simulink model "distr_obs_final"  (R2024b)
settings: Solver=VariableStepAuto  StartTime=0.0  StopTime=10  RelTol=1e-3
values from neighbouring files (symbols this model uses):
  A_sta = A-B*K    [main.m]
  Adj = [0,0,0,0,0,0 ... (first row only)    [chain_net.m]    (also in mesh_net.m = [0     3     1     1     1     1; star_net.m)
  C = [708.27 0]    [main.m]
  F = -F    [main.m]
  G = [1,0,0,0,0,0 ... (first row only)    [chain_net.m]    (also in mesh_net.m = diag([1,3,1,2,2,1]); star_net.m)
  noise_freq = 0.1    [main.m]
  noise_level = 10000    [main.m]
  x0 = [10, 1]    [main.m]
  x0_1 = [12 1]    [main.m]
  x0_2 = [4 1]    [main.m]
  x0_3 = [6 1]    [main.m]
  x0_4 = [6 1]    [main.m]
  x0_5 = [9 1]    [main.m]
  x0_6 = [8 1]    [main.m]
undefined symbols (not defined in the file or in its folder): maglev_dyn, observer
libraries: simulink x6
settings Model: Creator=Francesco  LastModifiedBy=filipnykvist

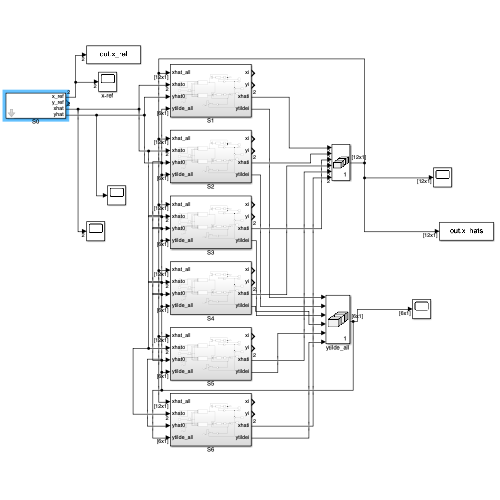
[thumbnail: Simulink's stored preview of the top-level diagram]
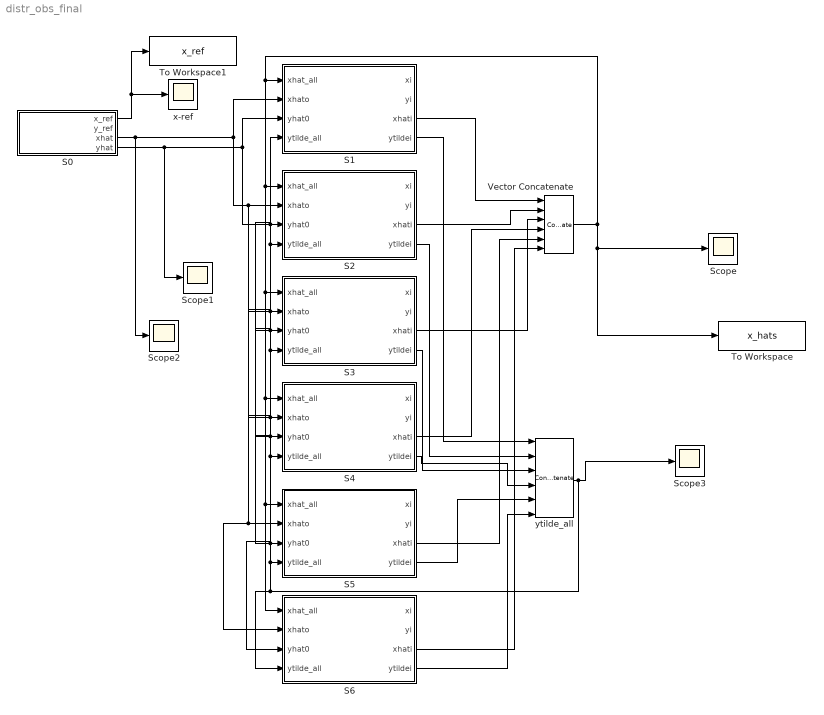
== system distr_obs_final ==
  S0 : Subsystem  mask{node_id=0}
      mask prompts: node_id "Nodo"
  S1 : Subsystem
  S2 : Subsystem
  S3 : Subsystem
  S4 : Subsystem
  S5 : Subsystem
  S6 : Subsystem
  Scope{,1..3} (4 alike) : Scope
  To Workspace : ToWorkspace  VariableName=x_hats  SaveFormat=Timeseries  SampleTime=-1
  To Workspace1 : ToWorkspace  VariableName=x_ref  SaveFormat=Timeseries  SampleTime=-1
  Vector Concatenate : Concatenate  NumInputs=6  Mode=Multidimensional array
  x-ref : Scope
  ytilde_all : Concatenate  NumInputs=6  Mode=Multidimensional array
  wires:
  Vector Concatenate/1 -> To Workspace/1, Scope/1, S6/1(xhat_all), S5/1(xhat_all), S4/1(xhat_all), S3/1(xhat_all), S2/1(xhat_all), S1/1(xhat_all)
  S0/3(xhat) -> Scope2/1, S2/2(xhato), S5/2(xhato), S6/2(xhato), S4/2(xhato), S3/2(xhato), S1/2(xhato)
  ytilde_all/1 -> S1/4(ytilde_all), S2/4(ytilde_all), S3/4(ytilde_all), S4/4(ytilde_all), S5/4(ytilde_all), S6/4(ytilde_all), Scope3/1
  S0/4(yhat) -> Scope1/1, S6/3(yhat0), S5/3(yhat0), S4/3(yhat0), S3/3(yhat0), S2/3(yhat0), S1/3(yhat0)
  S1/3(xhati) -> Vector Concatenate/1
  S2/3(xhati) -> Vector Concatenate/2
  S3/3(xhati) -> Vector Concatenate/3
  S4/3(xhati) -> Vector Concatenate/4
  S5/3(xhati) -> Vector Concatenate/5
  S6/3(xhati) -> Vector Concatenate/6
  S1/4(ytildei) -> ytilde_all/1
  S2/4(ytildei) -> ytilde_all/2
  S3/4(ytildei) -> ytilde_all/3
  S4/4(ytildei) -> ytilde_all/4
  S5/4(ytildei) -> ytilde_all/5
  S6/4(ytildei) -> ytilde_all/6
  S0/1(x_ref) -> x-ref/1, To Workspace1/1

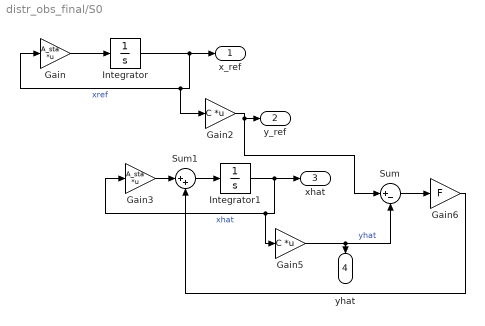
== system distr_obs_final/S0 ==
  Gain : Gain  Gain=A_sta  Multiplication=Matrix(K*u)
  Gain2 : Gain  Gain=C  Multiplication=Matrix(K*u)
  Gain3 : Gain  Gain=A_sta  Multiplication=Matrix(K*u)
  Gain5 : Gain  Gain=C  Multiplication=Matrix(K*u)
  Gain6 : Gain  Gain=F
  Integrator : Integrator  InitialCondition=x0
  Integrator1 : Integrator  InitialCondition=[0,0]'
  Sum : Sum  Inputs=|+-
  Sum1 : Sum  Inputs=|++
  x_ref : Outport
  y_ref : Outport  Port=2
  xhat : Outport  Port=3
  yhat : Outport  Port=4
  wires:
  Gain/1 -> Integrator/1
  Integrator/1 -> Gain/1, Gain2/1, x_ref/1  "xref"
  Gain2/1 -> Sum/1, y_ref/1
  Integrator1/1 -> Gain3/1, Gain5/1, xhat/1  "xhat"
  Gain5/1 -> yhat/1, Sum/2  "yhat"
  Sum/1 -> Gain6/1
  Gain3/1 -> Sum1/1
  Sum1/1 -> Integrator1/1
  Gain6/1 -> Sum1/2

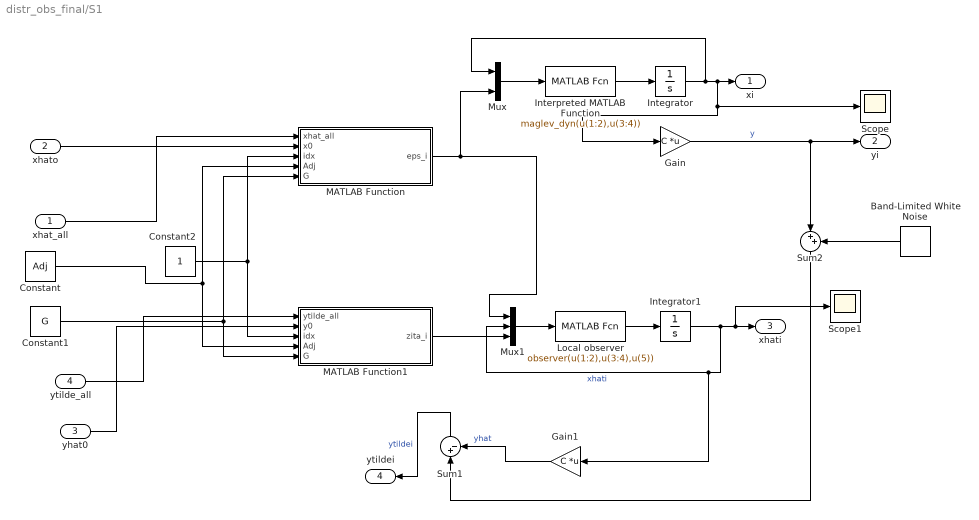
== system distr_obs_final/S1 ==
  xhat_all : Inport
  xhato : Inport  Port=2
  yhat0 : Inport  Port=3
  ytilde_all : Inport  Port=4
  Band-Limited White Noise : simulink/Sources/Band-Limited White Noise  Cov=[noise_level]  Ts=noise_freq  seed=[23341]
  Constant : Constant  Value=Adj
  Constant1 : Constant  Value=G
  Constant2 : Constant
  Gain : Gain  Gain=C  Multiplication=Matrix(K*u)
  Gain1 : Gain  Gain=C  Multiplication=Matrix(K*u)
  Integrator : Integrator  InitialCondition=x0_1
  Integrator1 : Integrator  InitialCondition=[0,0]'
  Interpreted MATLAB Function : MATLABFcn  MATLABFcn=maglev_dyn(u(1:2),u(3:4))
  Local observer : MATLABFcn  MATLABFcn=observer(u(1:2),u(3:4),u(5))  OutputDimensions=2
  MATLAB Function : MATLAB Function  TreatAsAtomicUnit=on
  MATLAB Function1 : MATLAB Function  TreatAsAtomicUnit=on
  Mux : Mux  Inputs=2
  Mux1 : Mux  Inputs=3
  Scope : Scope
  Scope1 : Scope
  Sum1 : Sum  Inputs=|+-
  Sum2 : Sum  Inputs=|++
  xi : Outport
  yi : Outport  Port=2
  xhati : Outport  Port=3
  ytildei : Outport  Port=4
  wires:
  Mux/1 -> Interpreted MATLAB Function/1
  Integrator/1 -> Mux/1, Scope/1, Gain/1, xi/1
  Interpreted MATLAB Function/1 -> Integrator/1
  Gain/1 -> Sum2/1, yi/1  "y"
  Local observer/1 -> Integrator1/1
  Integrator1/1 -> Mux1/2, Gain1/1, Scope1/1, xhati/1  "xhati"
  Gain1/1 -> Sum1/2  "yhat"
  Sum1/1 -> ytildei/1  "ytildei"
  xhat_all/1 -> MATLAB Function/1(xhat_all)
  Constant/1 -> MATLAB Function1/4(Adj), MATLAB Function/4(Adj)
  Constant1/1 -> MATLAB Function1/5(G), MATLAB Function/5(G)
  Constant2/1 -> MATLAB Function1/3(idx), MATLAB Function/3(idx)
  Mux1/1 -> Local observer/1
  MATLAB Function/1(eps_i) -> Mux/2, Mux1/1
  xhato/1 -> MATLAB Function/2(x0)
  Band-Limited White Noise/1 -> Sum2/2
  Sum2/1 -> Sum1/1
  MATLAB Function1/1(zita_i) -> Mux1/3
  ytilde_all/1 -> MATLAB Function1/1(ytilde_all)
  yhat0/1 -> MATLAB Function1/2(y0)

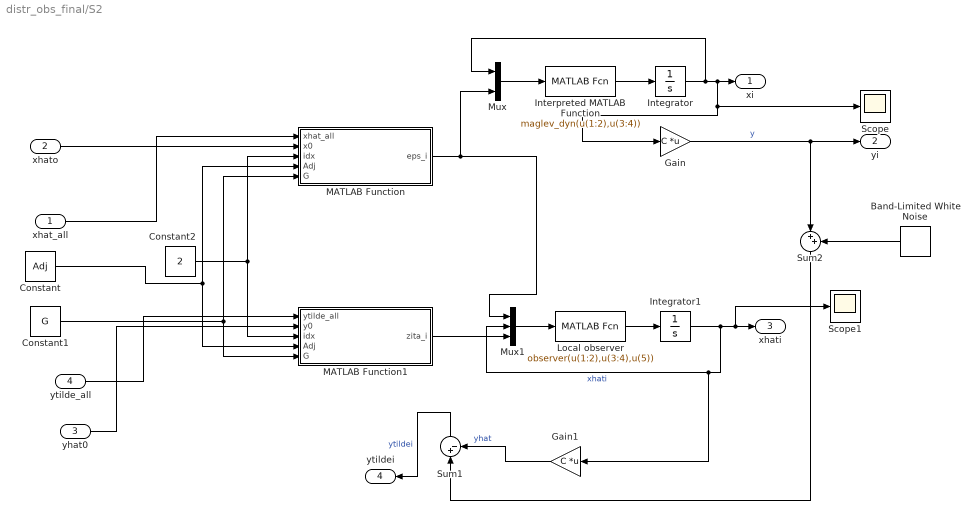
== system distr_obs_final/S2 ==
  xhat_all : Inport
  xhato : Inport  Port=2
  yhat0 : Inport  Port=3
  ytilde_all : Inport  Port=4
  Band-Limited White Noise : simulink/Sources/Band-Limited White Noise  Cov=[noise_level]  Ts=noise_freq  seed=[23341]
  Constant : Constant  Value=Adj
  Constant1 : Constant  Value=G
  Constant2 : Constant  Value=2
  Gain : Gain  Gain=C  Multiplication=Matrix(K*u)
  Gain1 : Gain  Gain=C  Multiplication=Matrix(K*u)
  Integrator : Integrator  InitialCondition=x0_2
  Integrator1 : Integrator  InitialCondition=[0,0]'
  Interpreted MATLAB Function : MATLABFcn  MATLABFcn=maglev_dyn(u(1:2),u(3:4))
  Local observer : MATLABFcn  MATLABFcn=observer(u(1:2),u(3:4),u(5))  OutputDimensions=2
  MATLAB Function : MATLAB Function  TreatAsAtomicUnit=on
  MATLAB Function1 : MATLAB Function  TreatAsAtomicUnit=on
  Mux : Mux  Inputs=2
  Mux1 : Mux  Inputs=3
  Scope : Scope
  Scope1 : Scope
  Sum1 : Sum  Inputs=|+-
  Sum2 : Sum  Inputs=|++
  xi : Outport
  yi : Outport  Port=2
  xhati : Outport  Port=3
  ytildei : Outport  Port=4
  wires:
  Mux/1 -> Interpreted MATLAB Function/1
  Integrator/1 -> Mux/1, Scope/1, Gain/1, xi/1
  Interpreted MATLAB Function/1 -> Integrator/1
  Gain/1 -> Sum2/1, yi/1  "y"
  Local observer/1 -> Integrator1/1
  Integrator1/1 -> Mux1/2, Gain1/1, Scope1/1, xhati/1  "xhati"
  Gain1/1 -> Sum1/2  "yhat"
  Sum1/1 -> ytildei/1  "ytildei"
  xhat_all/1 -> MATLAB Function/1(xhat_all)
  Constant/1 -> MATLAB Function1/4(Adj), MATLAB Function/4(Adj)
  Constant1/1 -> MATLAB Function1/5(G), MATLAB Function/5(G)
  Constant2/1 -> MATLAB Function1/3(idx), MATLAB Function/3(idx)
  Mux1/1 -> Local observer/1
  MATLAB Function/1(eps_i) -> Mux/2, Mux1/1
  xhato/1 -> MATLAB Function/2(x0)
  Band-Limited White Noise/1 -> Sum2/2
  Sum2/1 -> Sum1/1
  MATLAB Function1/1(zita_i) -> Mux1/3
  ytilde_all/1 -> MATLAB Function1/1(ytilde_all)
  yhat0/1 -> MATLAB Function1/2(y0)

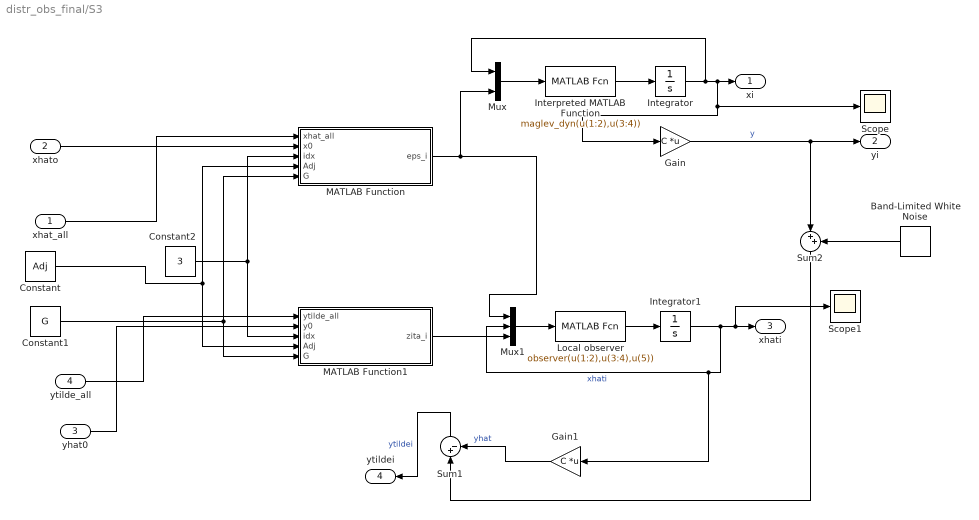
== system distr_obs_final/S3 ==
  xhat_all : Inport
  xhato : Inport  Port=2
  yhat0 : Inport  Port=3
  ytilde_all : Inport  Port=4
  Band-Limited White Noise : simulink/Sources/Band-Limited White Noise  Cov=[noise_level]  Ts=noise_freq  seed=[23341]
  Constant : Constant  Value=Adj
  Constant1 : Constant  Value=G
  Constant2 : Constant  Value=3
  Gain : Gain  Gain=C  Multiplication=Matrix(K*u)
  Gain1 : Gain  Gain=C  Multiplication=Matrix(K*u)
  Integrator : Integrator  InitialCondition=x0_3
  Integrator1 : Integrator  InitialCondition=[0,0]'
  Interpreted MATLAB Function : MATLABFcn  MATLABFcn=maglev_dyn(u(1:2),u(3:4))
  Local observer : MATLABFcn  MATLABFcn=observer(u(1:2),u(3:4),u(5))  OutputDimensions=2
  MATLAB Function : MATLAB Function  TreatAsAtomicUnit=on
  MATLAB Function1 : MATLAB Function  TreatAsAtomicUnit=on
  Mux : Mux  Inputs=2
  Mux1 : Mux  Inputs=3
  Scope : Scope
  Scope1 : Scope
  Sum1 : Sum  Inputs=|+-
  Sum2 : Sum  Inputs=|++
  xi : Outport
  yi : Outport  Port=2
  xhati : Outport  Port=3
  ytildei : Outport  Port=4
  wires:
  Mux/1 -> Interpreted MATLAB Function/1
  Integrator/1 -> Mux/1, Scope/1, Gain/1, xi/1
  Interpreted MATLAB Function/1 -> Integrator/1
  Gain/1 -> Sum2/1, yi/1  "y"
  Local observer/1 -> Integrator1/1
  Integrator1/1 -> Mux1/2, Gain1/1, Scope1/1, xhati/1  "xhati"
  Gain1/1 -> Sum1/2  "yhat"
  Sum1/1 -> ytildei/1  "ytildei"
  xhat_all/1 -> MATLAB Function/1(xhat_all)
  Constant/1 -> MATLAB Function1/4(Adj), MATLAB Function/4(Adj)
  Constant1/1 -> MATLAB Function1/5(G), MATLAB Function/5(G)
  Constant2/1 -> MATLAB Function1/3(idx), MATLAB Function/3(idx)
  Mux1/1 -> Local observer/1
  MATLAB Function/1(eps_i) -> Mux/2, Mux1/1
  xhato/1 -> MATLAB Function/2(x0)
  Band-Limited White Noise/1 -> Sum2/2
  Sum2/1 -> Sum1/1
  MATLAB Function1/1(zita_i) -> Mux1/3
  ytilde_all/1 -> MATLAB Function1/1(ytilde_all)
  yhat0/1 -> MATLAB Function1/2(y0)

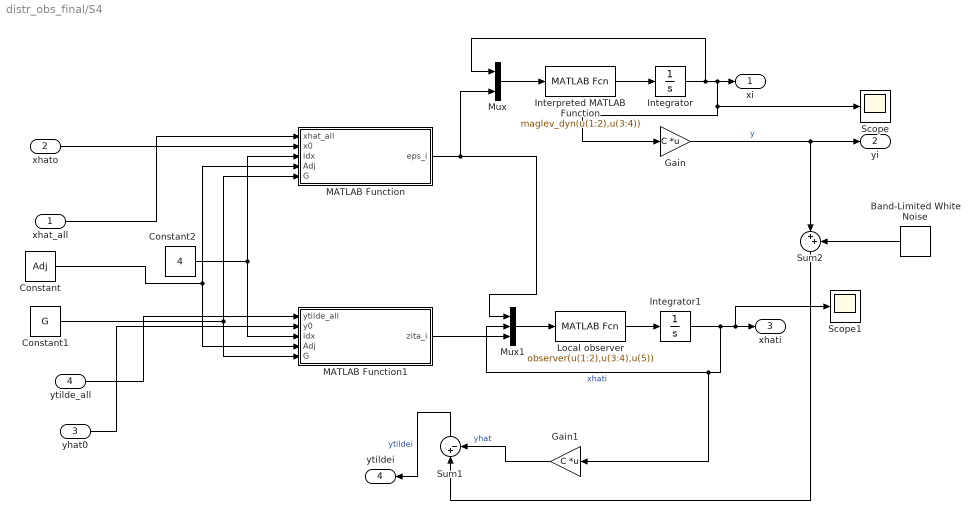
== system distr_obs_final/S4 ==
  xhat_all : Inport
  xhato : Inport  Port=2
  yhat0 : Inport  Port=3
  ytilde_all : Inport  Port=4
  Band-Limited White Noise : simulink/Sources/Band-Limited White Noise  Cov=[noise_level]  Ts=noise_freq  seed=[23341]
  Constant : Constant  Value=Adj
  Constant1 : Constant  Value=G
  Constant2 : Constant  Value=4
  Gain : Gain  Gain=C  Multiplication=Matrix(K*u)
  Gain1 : Gain  Gain=C  Multiplication=Matrix(K*u)
  Integrator : Integrator  InitialCondition=x0_4
  Integrator1 : Integrator  InitialCondition=[0,0]'
  Interpreted MATLAB Function : MATLABFcn  MATLABFcn=maglev_dyn(u(1:2),u(3:4))
  Local observer : MATLABFcn  MATLABFcn=observer(u(1:2),u(3:4),u(5))  OutputDimensions=2
  MATLAB Function : MATLAB Function  TreatAsAtomicUnit=on
  MATLAB Function1 : MATLAB Function  TreatAsAtomicUnit=on
  Mux : Mux  Inputs=2
  Mux1 : Mux  Inputs=3
  Scope : Scope
  Scope1 : Scope
  Sum1 : Sum  Inputs=|+-
  Sum2 : Sum  Inputs=|++
  xi : Outport
  yi : Outport  Port=2
  xhati : Outport  Port=3
  ytildei : Outport  Port=4
  wires:
  Mux/1 -> Interpreted MATLAB Function/1
  Integrator/1 -> Mux/1, Scope/1, Gain/1, xi/1
  Interpreted MATLAB Function/1 -> Integrator/1
  Gain/1 -> Sum2/1, yi/1  "y"
  Local observer/1 -> Integrator1/1
  Integrator1/1 -> Mux1/2, Gain1/1, Scope1/1, xhati/1  "xhati"
  Gain1/1 -> Sum1/2  "yhat"
  Sum1/1 -> ytildei/1  "ytildei"
  xhat_all/1 -> MATLAB Function/1(xhat_all)
  Constant/1 -> MATLAB Function1/4(Adj), MATLAB Function/4(Adj)
  Constant1/1 -> MATLAB Function1/5(G), MATLAB Function/5(G)
  Constant2/1 -> MATLAB Function1/3(idx), MATLAB Function/3(idx)
  Mux1/1 -> Local observer/1
  MATLAB Function/1(eps_i) -> Mux/2, Mux1/1
  xhato/1 -> MATLAB Function/2(x0)
  Band-Limited White Noise/1 -> Sum2/2
  Sum2/1 -> Sum1/1
  MATLAB Function1/1(zita_i) -> Mux1/3
  ytilde_all/1 -> MATLAB Function1/1(ytilde_all)
  yhat0/1 -> MATLAB Function1/2(y0)

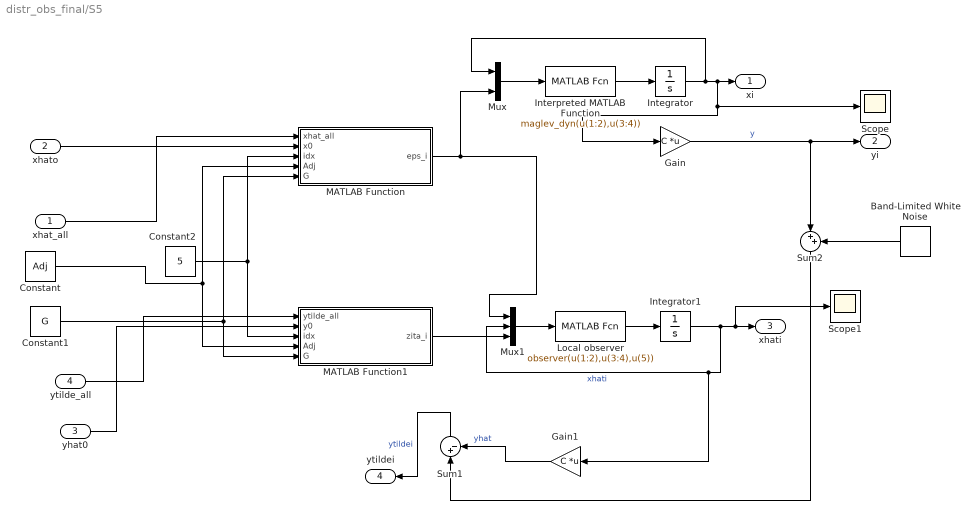
== system distr_obs_final/S5 ==
  xhat_all : Inport
  xhato : Inport  Port=2
  yhat0 : Inport  Port=3
  ytilde_all : Inport  Port=4
  Band-Limited White Noise : simulink/Sources/Band-Limited White Noise  Cov=[noise_level]  Ts=noise_freq  seed=[23341]
  Constant : Constant  Value=Adj
  Constant1 : Constant  Value=G
  Constant2 : Constant  Value=5
  Gain : Gain  Gain=C  Multiplication=Matrix(K*u)
  Gain1 : Gain  Gain=C  Multiplication=Matrix(K*u)
  Integrator : Integrator  InitialCondition=x0_5
  Integrator1 : Integrator  InitialCondition=[0,0]'
  Interpreted MATLAB Function : MATLABFcn  MATLABFcn=maglev_dyn(u(1:2),u(3:4))
  Local observer : MATLABFcn  MATLABFcn=observer(u(1:2),u(3:4),u(5))  OutputDimensions=2
  MATLAB Function : MATLAB Function  TreatAsAtomicUnit=on
  MATLAB Function1 : MATLAB Function  TreatAsAtomicUnit=on
  Mux : Mux  Inputs=2
  Mux1 : Mux  Inputs=3
  Scope : Scope
  Scope1 : Scope
  Sum1 : Sum  Inputs=|+-
  Sum2 : Sum  Inputs=|++
  xi : Outport
  yi : Outport  Port=2
  xhati : Outport  Port=3
  ytildei : Outport  Port=4
  wires:
  Mux/1 -> Interpreted MATLAB Function/1
  Integrator/1 -> Mux/1, Scope/1, Gain/1, xi/1
  Interpreted MATLAB Function/1 -> Integrator/1
  Gain/1 -> Sum2/1, yi/1  "y"
  Local observer/1 -> Integrator1/1
  Integrator1/1 -> Mux1/2, Gain1/1, Scope1/1, xhati/1  "xhati"
  Gain1/1 -> Sum1/2  "yhat"
  Sum1/1 -> ytildei/1  "ytildei"
  xhat_all/1 -> MATLAB Function/1(xhat_all)
  Constant/1 -> MATLAB Function1/4(Adj), MATLAB Function/4(Adj)
  Constant1/1 -> MATLAB Function1/5(G), MATLAB Function/5(G)
  Constant2/1 -> MATLAB Function1/3(idx), MATLAB Function/3(idx)
  Mux1/1 -> Local observer/1
  MATLAB Function/1(eps_i) -> Mux/2, Mux1/1
  xhato/1 -> MATLAB Function/2(x0)
  Band-Limited White Noise/1 -> Sum2/2
  Sum2/1 -> Sum1/1
  MATLAB Function1/1(zita_i) -> Mux1/3
  ytilde_all/1 -> MATLAB Function1/1(ytilde_all)
  yhat0/1 -> MATLAB Function1/2(y0)

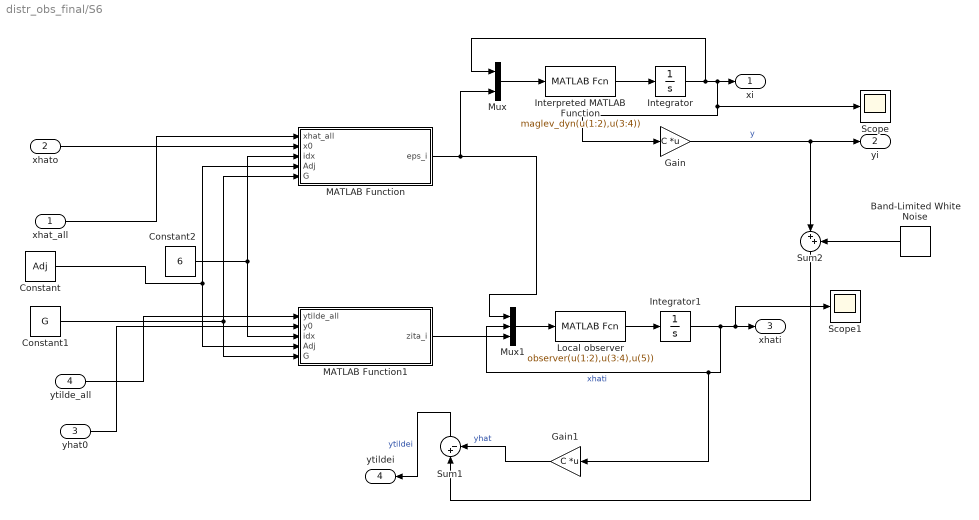
== system distr_obs_final/S6 ==
  xhat_all : Inport
  xhato : Inport  Port=2
  yhat0 : Inport  Port=3
  ytilde_all : Inport  Port=4
  Band-Limited White Noise : simulink/Sources/Band-Limited White Noise  Cov=[noise_level]  Ts=noise_freq  seed=[23341]
  Constant : Constant  Value=Adj
  Constant1 : Constant  Value=G
  Constant2 : Constant  Value=6
  Gain : Gain  Gain=C  Multiplication=Matrix(K*u)
  Gain1 : Gain  Gain=C  Multiplication=Matrix(K*u)
  Integrator : Integrator  InitialCondition=x0_6
  Integrator1 : Integrator  InitialCondition=[0,0]'
  Interpreted MATLAB Function : MATLABFcn  MATLABFcn=maglev_dyn(u(1:2),u(3:4))
  Local observer : MATLABFcn  MATLABFcn=observer(u(1:2),u(3:4),u(5))  OutputDimensions=2
  MATLAB Function : MATLAB Function  TreatAsAtomicUnit=on
  MATLAB Function1 : MATLAB Function  TreatAsAtomicUnit=on
  Mux : Mux  Inputs=2
  Mux1 : Mux  Inputs=3
  Scope : Scope
  Scope1 : Scope
  Sum1 : Sum  Inputs=|+-
  Sum2 : Sum  Inputs=|++
  xi : Outport
  yi : Outport  Port=2
  xhati : Outport  Port=3
  ytildei : Outport  Port=4
  wires:
  Mux/1 -> Interpreted MATLAB Function/1
  Integrator/1 -> Mux/1, Scope/1, Gain/1, xi/1
  Interpreted MATLAB Function/1 -> Integrator/1
  Gain/1 -> Sum2/1, yi/1  "y"
  Local observer/1 -> Integrator1/1
  Integrator1/1 -> Mux1/2, Gain1/1, Scope1/1, xhati/1  "xhati"
  Gain1/1 -> Sum1/2  "yhat"
  Sum1/1 -> ytildei/1  "ytildei"
  xhat_all/1 -> MATLAB Function/1(xhat_all)
  Constant/1 -> MATLAB Function1/4(Adj), MATLAB Function/4(Adj)
  Constant1/1 -> MATLAB Function1/5(G), MATLAB Function/5(G)
  Constant2/1 -> MATLAB Function1/3(idx), MATLAB Function/3(idx)
  Mux1/1 -> Local observer/1
  MATLAB Function/1(eps_i) -> Mux/2, Mux1/1
  xhato/1 -> MATLAB Function/2(x0)
  Band-Limited White Noise/1 -> Sum2/2
  Sum2/1 -> Sum1/1
  MATLAB Function1/1(zita_i) -> Mux1/3
  ytilde_all/1 -> MATLAB Function1/1(ytilde_all)
  yhat0/1 -> MATLAB Function1/2(y0)

== matlab function distr_obs_final/S2/MATLAB Function ==
  data: xhat_all input; eps_i output; x0 input; idx input; Adj input; G input
function eps_i = calcola_epsilon(xhat_all, x0, idx, Adj, G)
    
    a_row = Adj(idx, :);
    g_row = G(idx, :);

    % Assicurazione che i vettori siano nelle giuste forme  
    x0 = x0(:);            
    xhat_all = xhat_all(:); 

    % Selezione del blocco 2x1 corrente
    idx_i = 2 * idx - 1;                      
    xhat_i = xhat_all(idx_i : idx_i + 1);      
                 
    g_i = g_row(idx);                      

    % Dimensioni
    nCols = length(a_row); % nCols = 6
    
    % Inizializzazione matrice estesa a blocchi
    a_row_expand = zeros(2, 2 * nCols); % 2x12

    % Costruzione della matrixe estesa
    for c = 1 : nCols 
        val = a_row(1, c);
        colPos = 2 * c - 1;
        if val ~= 0
            a_row_expand(:, colPos:colPos+1) = val * eye(2);
        end
    end

    % Differenze
    xdiff = xhat_all - repmat(xhat_i, nCols, 1);  
    xdiff = reshape(xdiff, 12, 1);                 
    diff_ref = x0 - xhat_i;                      

    % Calcolo eps_i
    eps_i = a_row_expand * xdiff + g_i * diff_ref;  % 2x1
end

== matlab function distr_obs_final/S5/MATLAB Function1 ==
  data: ytilde_all input; zita_i output; y0 input; idx input; Adj input; G input
function zita_i = calcola_zita(ytilde_all, y0, idx, Adj, G)
    % Get adjacency and pinning row for agent i.
    a_row = Adj(idx, :);
    g_i = G(idx, idx);  

    % Extract ytilde_i.
    ytilde_i = ytilde_all(idx);

    % Compute the difference to each neighbor.
    ydiff = ytilde_all - ytilde_i;  % 6x1 vector of differences

    % Weighted sum of neighbor differences.
    sum_neighbors = a_row * ydiff;  % scalar

    % Leader (reference) difference.
    diff_ref = y0 - ytilde_i;       % scalar

    % Combine to form zita_i.
    zita_i = sum_neighbors + g_i * diff_ref;  % scalar
end

== matlab function distr_obs_final/S6/MATLAB Function ==
  data: xhat_all input; eps_i output; x0 input; idx input; Adj input; G input
function eps_i = calcola_epsilon(xhat_all, x0, idx, Adj, G)
    
    a_row = Adj(idx, :);
    g_row = G(idx, :);

    % Assicurazione che i vettori siano nelle giuste forme  
    x0 = x0(:);            
    xhat_all = xhat_all(:); 

    % Selezione del blocco 2x1 corrente
    idx_i = 2 * idx - 1;                      
    xhat_i = xhat_all(idx_i : idx_i + 1);      
                 
    g_i = g_row(idx);                      

    % Dimensioni
    nCols = length(a_row); % nCols = 6
    
    % Inizializzazione matrice estesa a blocchi
    a_row_expand = zeros(2, 2 * nCols); % 2x12

    % Costruzione della matrixe estesa
    for c = 1 : nCols 
        val = a_row(1, c);
        colPos = 2 * c - 1;
        if val ~= 0
            a_row_expand(:, colPos:colPos+1) = val * eye(2);
        end
    end

    % Differenze
    xdiff = xhat_all - repmat(xhat_i, nCols, 1);  
    xdiff = reshape(xdiff, 12, 1);                 
    diff_ref = x0 - xhat_i;                      

    % Calcolo eps_i
    eps_i = a_row_expand * xdiff + g_i * diff_ref;  % 2x1
end

== matlab function distr_obs_final/S6/MATLAB Function1 ==
  data: ytilde_all input; zita_i output; y0 input; idx input; Adj input; G input
function zita_i = calcola_zita(ytilde_all, y0, idx, Adj, G)
    % Get adjacency and pinning row for agent i.
    a_row = Adj(idx, :);
    g_i = G(idx, idx); 

    % Extract ytilde_i.
    ytilde_i = ytilde_all(idx);

    % Compute the difference to each neighbor.
    ydiff = ytilde_all - ytilde_i;  % 6x1 vector of differences

    % Weighted sum of neighbor differences.
    sum_neighbors = a_row * ydiff;  % scalar

    % Leader (reference) difference.
    diff_ref = y0 - ytilde_i;       % scalar

    % Combine to form zita_i.
    zita_i = sum_neighbors + g_i * diff_ref;  % scalar
end

== matlab function distr_obs_final/S1/MATLAB Function ==
  data: xhat_all input; eps_i output; x0 input; idx input; Adj input; G input
function eps_i = calcola_epsilon(xhat_all, x0, idx, Adj, G)
    
    a_row = Adj(idx, :);
    g_row = G(idx, :);

    % Assicurazione che i vettori siano nelle giuste forme  
    x0 = x0(:);            
    xhat_all = xhat_all(:); 

    % Selezione del blocco 2x1 corrente
    idx_i = 2 * idx - 1;                      
    xhat_i = xhat_all(idx_i : idx_i + 1);      
                 
    g_i = g_row(idx);                      

    % Dimensioni
    nCols = length(a_row); % nCols = 6
    
    % Inizializzazione matrice estesa a blocchi
    a_row_expand = zeros(2, 2 * nCols); % 2x12

    % Costruzione della matrixe estesa
    for c = 1 : nCols 
        val = a_row(1, c);
        colPos = 2 * c - 1;
        if val ~= 0
            a_row_expand(:, colPos:colPos+1) = val * eye(2);
        end
    end

    % Differenze
    xdiff = xhat_all - repmat(xhat_i, nCols, 1);  
    xdiff = reshape(xdiff, 12, 1);                 
    diff_ref = x0 - xhat_i;                      

    % Calcolo eps_i
    eps_i = a_row_expand * xdiff + g_i * diff_ref;  % 2x1
end

== matlab function distr_obs_final/S2/MATLAB Function1 ==
  data: ytilde_all input; zita_i output; y0 input; idx input; Adj input; G input
function zita_i = calcola_zita(ytilde_all, y0, idx, Adj, G)
    % Get adjacency and pinning row for agent i.
    a_row = Adj(idx, :);
    g_i = G(idx, idx);

    % Extract ytilde_i.
    ytilde_i = ytilde_all(idx);

    % Compute the difference to each neighbor.
    ydiff = ytilde_all - ytilde_i;  % 6x1 vector of differences

    % Weighted sum of neighbor differences.
    sum_neighbors = a_row * ydiff;  % scalar

    % Leader (reference) difference.
    diff_ref = y0 - ytilde_i;       % scalar

    % Combine to form zita_i.
    zita_i = sum_neighbors + g_i * diff_ref;  % scalar
end

== matlab function distr_obs_final/S3/MATLAB Function ==
  data: xhat_all input; eps_i output; x0 input; idx input; Adj input; G input
function eps_i = calcola_epsilon(xhat_all, x0, idx, Adj, G)
    
    a_row = Adj(idx, :);
    g_row = G(idx, :);

    % Assicurazione che i vettori siano nelle giuste forme  
    x0 = x0(:);            
    xhat_all = xhat_all(:); 

    % Selezione del blocco 2x1 corrente
    idx_i = 2 * idx - 1;                      
    xhat_i = xhat_all(idx_i : idx_i + 1);      
                 
    g_i = g_row(idx);                      

    % Dimensioni
    nCols = length(a_row); % nCols = 6
    
    % Inizializzazione matrice estesa a blocchi
    a_row_expand = zeros(2, 2 * nCols); % 2x12

    % Costruzione della matrixe estesa
    for c = 1 : nCols 
        val = a_row(1, c);
        colPos = 2 * c - 1;
        if val ~= 0
            a_row_expand(:, colPos:colPos+1) = val * eye(2);
        end
    end

    % Differenze
    xdiff = xhat_all - repmat(xhat_i, nCols, 1);  
    xdiff = reshape(xdiff, 12, 1);                 
    diff_ref = x0 - xhat_i;                      

    % Calcolo eps_i
    eps_i = a_row_expand * xdiff + g_i * diff_ref;  % 2x1
end

== matlab function distr_obs_final/S3/MATLAB Function1 ==
  data: ytilde_all input; zita_i output; y0 input; idx input; Adj input; G input
function zita_i = calcola_zita(ytilde_all, y0, idx, Adj, G)
    % Get adjacency and pinning row for agent i.
    a_row = Adj(idx, :);
    g_i = G(idx, idx);

    % Extract ytilde_i.
    ytilde_i = ytilde_all(idx);

    % Compute the difference to each neighbor.
    ydiff = ytilde_all - ytilde_i;  % 6x1 vector of differences

    % Weighted sum of neighbor differences.
    sum_neighbors = a_row * ydiff;  % scalar

    % Leader (reference) difference.
    diff_ref = y0 - ytilde_i;       % scalar

    % Combine to form zita_i.
    zita_i = sum_neighbors + g_i * diff_ref;  % scalar
end

== matlab function distr_obs_final/S4/MATLAB Function ==
  data: xhat_all input; eps_i output; x0 input; idx input; Adj input; G input
function eps_i = calcola_epsilon(xhat_all, x0, idx, Adj, G)
    
    a_row = Adj(idx, :);
    g_row = G(idx, :);

    % Assicurazione che i vettori siano nelle giuste forme  
    x0 = x0(:);            
    xhat_all = xhat_all(:); 

    % Selezione del blocco 2x1 corrente
    idx_i = 2 * idx - 1;                      
    xhat_i = xhat_all(idx_i : idx_i + 1);      
                 
    g_i = g_row(idx);                      

    % Dimensioni
    nCols = length(a_row); % nCols = 6
    
    % Inizializzazione matrice estesa a blocchi
    a_row_expand = zeros(2, 2 * nCols); % 2x12

    % Costruzione della matrixe estesa
    for c = 1 : nCols 
        val = a_row(1, c);
        colPos = 2 * c - 1;
        if val ~= 0
            a_row_expand(:, colPos:colPos+1) = val * eye(2);
        end
    end

    % Differenze
    xdiff = xhat_all - repmat(xhat_i, nCols, 1);  
    xdiff = reshape(xdiff, 12, 1);                 
    diff_ref = x0 - xhat_i;                      

    % Calcolo eps_i
    eps_i = a_row_expand * xdiff + g_i * diff_ref;  % 2x1
end

== matlab function distr_obs_final/S1/MATLAB Function1 ==
  data: ytilde_all input; zita_i output; y0 input; idx input; Adj input; G input
function zita_i = calcola_zita(ytilde_all, y0, idx, Adj, G)
    % Get adjacency and pinning row for agent i.
    a_row = Adj(idx, :);
    g_i = G(idx, idx);

    % Extract ytilde_i.
    ytilde_i = ytilde_all(idx);

    % Compute the difference to each neighbor.
    ydiff = ytilde_all - ytilde_i;  % 6x1 vector of differences

    % Weighted sum of neighbor differences.
    sum_neighbors = a_row * ydiff;  % scalar

    % Leader (reference) difference.
    diff_ref = y0 - ytilde_i;       % scalar

    % Combine to form zita_i.
    zita_i = sum_neighbors + g_i * diff_ref;  % scalar
end

== matlab function distr_obs_final/S4/MATLAB Function1 ==
  data: ytilde_all input; zita_i output; y0 input; idx input; Adj input; G input
function zita_i = calcola_zita(ytilde_all, y0, idx, Adj, G)
    % Get adjacency and pinning row for agent i.
    a_row = Adj(idx, :);
    g_i = G(idx, idx);

    % Extract ytilde_i.
    ytilde_i = ytilde_all(idx);

    % Compute the difference to each neighbor.
    ydiff = ytilde_all - ytilde_i;  % 6x1 vector of differences

    % Weighted sum of neighbor differences.
    sum_neighbors = a_row * ydiff;  % scalar

    % Leader (reference) difference.
    diff_ref = y0 - ytilde_i;       % scalar

    % Combine to form zita_i.
    zita_i = sum_neighbors + g_i * diff_ref;  % scalar
end

== matlab function distr_obs_final/S5/MATLAB Function ==
  data: xhat_all input; eps_i output; x0 input; idx input; Adj input; G input
function eps_i = calcola_epsilon(xhat_all, x0, idx, Adj, G)
    
    a_row = Adj(idx, :);
    g_row = G(idx, :);

    % Assicurazione che i vettori siano nelle giuste forme  
    x0 = x0(:);            
    xhat_all = xhat_all(:); 

    % Selezione del blocco 2x1 corrente
    idx_i = 2 * idx - 1;                      
    xhat_i = xhat_all(idx_i : idx_i + 1);      
                 
    g_i = g_row(idx);                      

    % Dimensioni
    nCols = length(a_row); % nCols = 6
    
    % Inizializzazione matrice estesa a blocchi
    a_row_expand = zeros(2, 2 * nCols); % 2x12

    % Costruzione della matrixe estesa
    for c = 1 : nCols 
        val = a_row(1, c);
        colPos = 2 * c - 1;
        if val ~= 0
            a_row_expand(:, colPos:colPos+1) = val * eye(2);
        end
    end

    % Differenze
    xdiff = xhat_all - repmat(xhat_i, nCols, 1);  
    xdiff = reshape(xdiff, 12, 1);                 
    diff_ref = x0 - xhat_i;                      

    % Calcolo eps_i
    eps_i = a_row_expand * xdiff + g_i * diff_ref;  % 2x1
end
